simulink model "AutonomousDrivingACC"  (R2023a)
settings: Solver=ode45  StartTime=0.0  StopTime=StopTime_s  RelTol=1e-3
model workspace (MAT data in the model file):
  DesiredGap_m = 25
  DragCoeff = 0.05
  EgoInitialPos_m = 0
  EgoInitialSpeed_mps = 0
  KdRelativeSpeed = 0.5
  KpGap = 0.1
  LeadInitialPos_m = 60
  LeadSpeed_mps = 20
  StopTime_s = 60
settings Model: Creator=LZH  LastModifiedBy=LZH

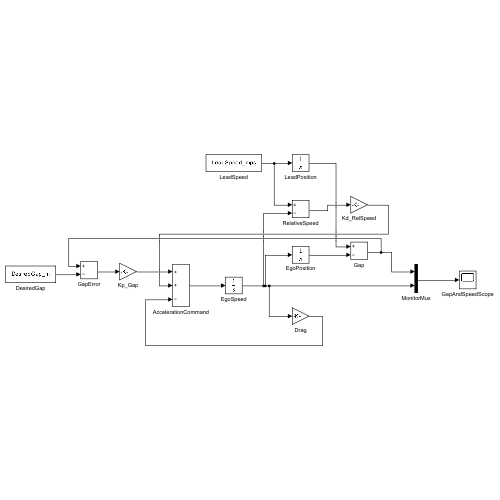
[thumbnail: Simulink's stored preview of the top-level diagram]
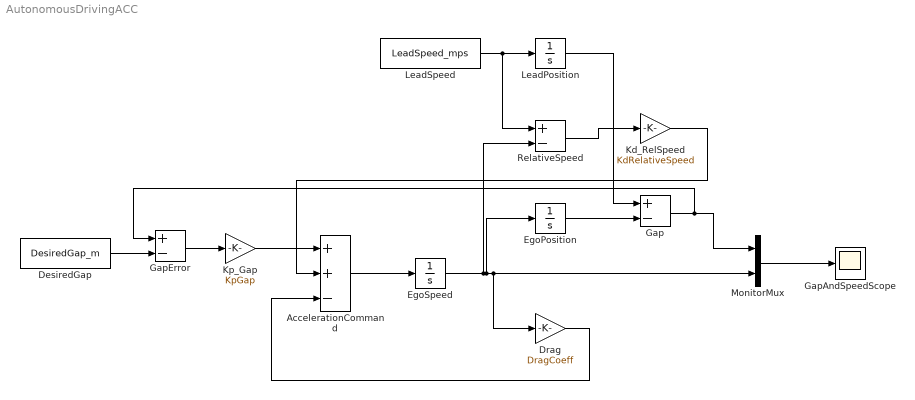
== system AutonomousDrivingACC ==
  AccelerationCommand : Sum  Inputs=++-
  DesiredGap : Constant  Value=DesiredGap_m
  Drag : Gain  Gain=DragCoeff
  EgoPosition : Integrator  InitialCondition=EgoInitialPos_m
  EgoSpeed : Integrator  InitialCondition=EgoInitialSpeed_mps
  Gap : Sum  Inputs=+-
  GapAndSpeedScope : Scope
  GapError : Sum  Inputs=+-
  Kd_RelSpeed : Gain  Gain=KdRelativeSpeed
  Kp_Gap : Gain  Gain=KpGap
  LeadPosition : Integrator  InitialCondition=LeadInitialPos_m
  LeadSpeed : Constant  Value=LeadSpeed_mps
  MonitorMux : Mux  Inputs=2
  RelativeSpeed : Sum  Inputs=+-
  wires:
  MonitorMux/1 -> GapAndSpeedScope/1
  AccelerationCommand/1 -> EgoSpeed/1
  Drag/1 -> AccelerationCommand/3
  Kd_RelSpeed/1 -> AccelerationCommand/2
  Kp_Gap/1 -> AccelerationCommand/1
  RelativeSpeed/1 -> Kd_RelSpeed/1
  GapError/1 -> Kp_Gap/1
  DesiredGap/1 -> GapError/2
  Gap/1 -> MonitorMux/1, GapError/1
  EgoPosition/1 -> Gap/2
  EgoSpeed/1 -> MonitorMux/2, Drag/1, EgoPosition/1, RelativeSpeed/2
  LeadPosition/1 -> Gap/1
  LeadSpeed/1 -> RelativeSpeed/1, LeadPosition/1
